simulink model "getDataFromXplane"  (R2018a)
settings: Solver=VariableStepAuto  StartTime=0.0  StopTime=inf  RelTol=1e-3
libraries: etargetslib x1, sldrtlib x1, dspnetwork x1
settings Model: Creator=Flight Test Lab  LastModifiedBy=Flight Test Lab

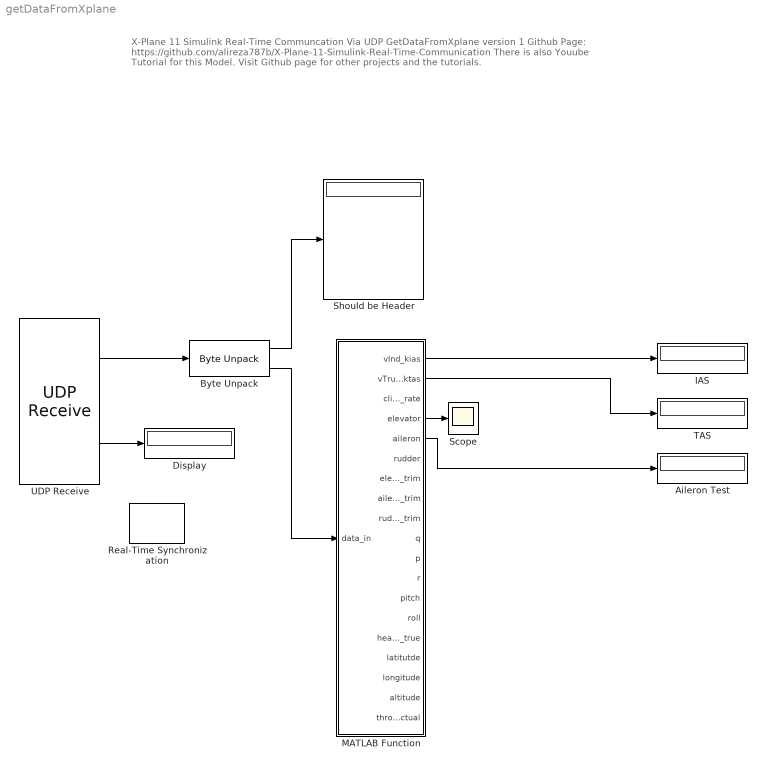
== system getDataFromXplane ==
  note: X-Plane 11 Simulink Real-Time Communcation Via UDP
      | GetDataFromXplane version 1
      | Github Page:
      | https://github.com/alireza787b/X-Plane-11-Simulink-Real-Time-Communication
      | There is also Youube Tutorial for this Model.
      | Visit Github page for other projects and the tutorials.
  Aileron Test : Display
  Byte Unpack : etargetslib/Byte Unpack  dimensions={5,[9,8]}  datatypes={'uint8','single'}  byteAlign=1
  Display : Display
  IAS : Display
  MATLAB Function : MATLAB Function  TreatAsAtomicUnit=on
  Real-Time Synchronization : sldrtlib/Real-Time Synchronization  SampleTime=0.1  MaxMissedTicks=10  ShowMissedTicks=off  YieldWhenWaiting=off
  Scope : Scope
  Should be Header : Display
  TAS : Display
  UDP Receive : dspnetwork/UDP Receive  localURL='0.0.0.0'  localPort=49004  remoteURL='127.0.0.1'  remotePort=-1  recvBufferSize=8192  dims=293  signalDatatype=uint8  isVarSize=off  showBlockingTime=off  blockingTime=0  sampletime=inf  blockPlatform=[]
      settings: SourceProductName=DSP System Toolbox  SourceProductBaseCode=DS
  wires:
  Byte Unpack/2 -> MATLAB Function/1(data_in)
  Byte Unpack/1 -> Should be Header/1
  UDP Receive/1 -> Byte Unpack/1
  MATLAB Function/5(aileron) -> Aileron Test/1
  UDP Receive/2 -> Display/1
  MATLAB Function/2(vTrue_ktas) -> TAS/1
  MATLAB Function/4(elevator) -> Scope/1
  MATLAB Function/1(vInd_kias) -> IAS/1

== matlab function getDataFromXplane/MATLAB Function ==
  data: data_in input; vInd_kias output; vTrue_ktas output; climb_rate output; elevator output; aileron output; rudder output; elevator_trim output; aileron_trim output; rudder_trim output; q output; p output; r output; pitch output; roll output; heading_true output; latitutde output; longitude output; altitude output; throttle_actual output
function [vInd_kias,vTrue_ktas,...
    climb_rate,...
    elevator,aileron,rudder,...
    elevator_trim,aileron_trim,rudder_trim,...
    q,p,r,...
    pitch, roll, heading_true,...
    latitutde, longitude, altitude,...
    throttle_actual] = decoder(data_in)
 vInd_kias = data_in(2,1);
 vTrue_ktas = data_in(4,1);
 climb_rate = data_in(4,2);
 elevator = data_in(2,3);
 aileron = data_in(3,3);
 rudder= data_in(4,3);
 elevator_trim= data_in(2,4);
 aileron_trim= data_in(3,4);
 rudder_trim= data_in(4,4);
 q= data_in(2,5);
 p= data_in(3,5);
 r= data_in(4,5);
 pitch= data_in(2,6);
 roll= data_in(3,6);
 heading_true= data_in(4,6);
 latitutde= data_in(2,7);
 longitude= data_in(3,7);
 altitude= data_in(4,7);
 throttle_actual = data_in(2,8);
end
